simulink library "IdealMagnetorquer"  (R2020b)
settings: Solver=VariableStepAuto  StartTime=0.0  StopTime=10.0  RelTol=1e-3
libraries: sharedutil x1
settings Model: Creator=dbell44  LastModifiedBy=dbell44

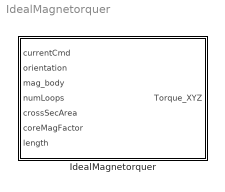
== system IdealMagnetorquer ==
  IdealMagnetorquer : Subsystem

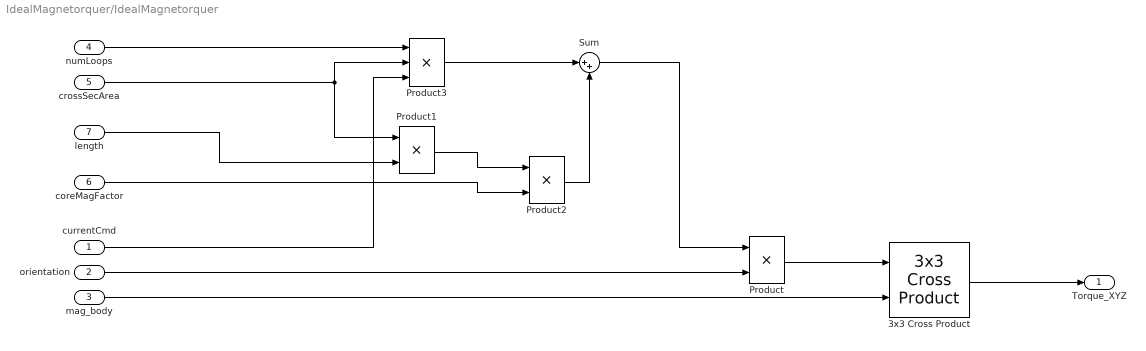
== system IdealMagnetorquer/IdealMagnetorquer ==
  currentCmd : Inport
  orientation : Inport  Port=2
  mag_body : Inport  Port=3
  numLoops : Inport  Port=4
  crossSecArea : Inport  Port=5
  coreMagFactor : Inport  Port=6
  length : Inport  Port=7
  3x3 Cross Product : sharedutil/3x3 Cross Product  aMode=aMode
      settings: SourceProductBaseCode=AE,PW,MT,UV,VE,VP
  Product : Product
  Product1 : Product
  Product2 : Product
  Product3 : Product  Inputs=3
  Sum : Sum  Inputs=|++
  Torque_XYZ : Outport
  wires:
  currentCmd/1 -> Product3/3
  orientation/1 -> Product/2
  Product/1 -> 3x3 Cross Product/1
  mag_body/1 -> 3x3 Cross Product/2
  3x3 Cross Product/1 -> Torque_XYZ/1
  crossSecArea/1 -> Product1/1, Product3/2
  length/1 -> Product1/2
  Product1/1 -> Product2/1
  coreMagFactor/1 -> Product2/2
  numLoops/1 -> Product3/1
  Product3/1 -> Sum/1
  Product2/1 -> Sum/2
  Sum/1 -> Product/1
